simulink model "Quadruple_Tank_Simu_Model"  (R2021b)
settings: Solver=VariableStepAuto  StartTime=0.0  StopTime=300  FixedStep=1  RelTol=1e-3
values from neighbouring files (symbols this model uses):
  a1 = 0.17795237427    [Dados_Tanques.mat]    (also in double_tank_simu.m)
  A1 = 15.5179165474    [Dados_Tanques.mat]    (also in double_tank_simu.m)
  a2 = 0.17795237427    [Dados_Tanques.mat]    (also in double_tank_simu.m)
  A2 = 15.5179165474    [Dados_Tanques.mat]    (also in double_tank_simu.m)
  g = 981    [Dados_Tanques.mat]    (also in double_tank_simu.m)
  x1eq = 15    [Dados_Tanques.mat]    (also in double_tank_simu.m = (1/(2*g))*((km*ueq)/a1)^2)
  x2eq = 15    [Dados_Tanques.mat]    (also in double_tank_simu.m)
undefined symbols (not defined in the file or in its folder): a3, A3, a4, A4, k1, k2, q1, q2, u1eq, u2eq, x3eq, x4eq
libraries: instrumentlib x2
settings Model: Creator=mathe  LastModifiedBy=mathe

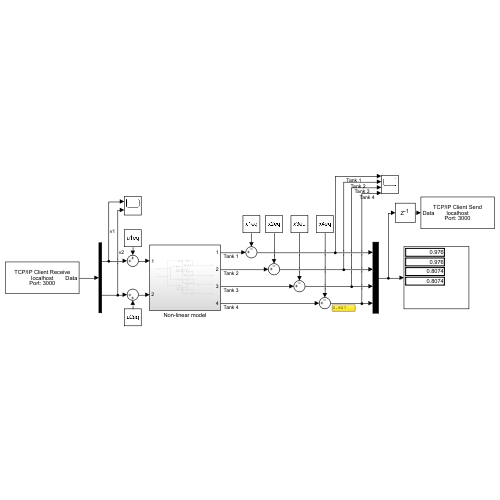
[thumbnail: Simulink's stored preview of the top-level diagram]
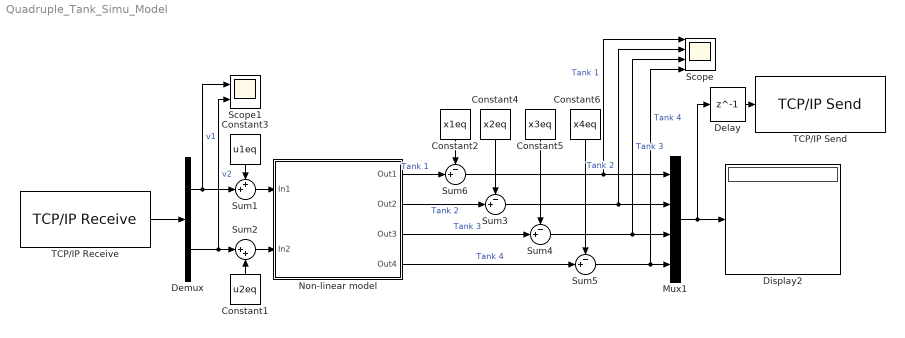
== system Quadruple_Tank_Simu_Model ==
  Constant1 : Constant  Value=u2eq
  Constant2 : Constant  Value=x1eq
  Constant3 : Constant  Value=u1eq
  Constant4 : Constant  Value=x2eq
  Constant5 : Constant  Value=x3eq
  Constant6 : Constant  Value=x4eq
  Delay : Delay  DelayLength=1  InitialCondition=0
  Demux : Demux  Outputs=2
  Display2 : Display
  Mux1 : Mux
  Non-linear model : Subsystem
  Scope : Scope  NumInputPorts=4
  Scope1 : Scope  NumInputPorts=2
  Sum1 : Sum  Inputs=++|
  Sum2 : Sum  Inputs=|++
  Sum{3..6} (4 alike) : Sum  Inputs=-+|
  TCP/IP Receive : instrumentlib/TCP//IP Receive  Priority=2  Host=localhost  Port=3000  DataSize=[ 2, 1 ]  DataType=double  ASCIIFormatting=%f  Terminator=LF  CustomTerminator=10  ByteOrder=big-endian  EnableBlockingMode=on  Timeout=300  SampleTime=1  SimulateUsing=Interpreted execution
  TCP/IP Send : instrumentlib/TCP//IP Send  Priority=1  Host=localhost  Port=3000  ByteOrder=big-endian  EnableBlockingMode=on  Timeout=300  TransferDelay=off  SimulateUsing=Interpreted execution
  wires:
  Non-linear model/1(Out1) -> Sum6/2  "Tank 1"
  Constant3/1 -> Sum1/1
  Sum1/1 -> Non-linear model/1(In1)
  Sum2/1 -> Non-linear model/2(In2)
  Constant1/1 -> Sum2/2
  Sum6/1 -> Scope/1, Mux1/1  "Tank 1"
  Constant2/1 -> Sum6/1
  Sum3/1 -> Scope/2, Mux1/2  "Tank 2"
  Non-linear model/2(Out2) -> Sum3/2  "Tank 2"
  Constant4/1 -> Sum3/1
  Sum5/1 -> Scope/4, Mux1/4  "Tank 4"
  Non-linear model/4(Out4) -> Sum5/2  "Tank 4"
  Non-linear model/3(Out3) -> Sum4/2  "Tank 3"
  Sum4/1 -> Scope/3, Mux1/3  "Tank 3"
  Constant5/1 -> Sum4/1
  Constant6/1 -> Sum5/1
  Demux/1 -> Scope1/1, Sum1/2  "v1"
  Demux/2 -> Scope1/2, Sum2/1  "v2"
  Mux1/1 -> Delay/1, Display2/1
  TCP/IP Receive/1 -> Demux/1
  Delay/1 -> TCP/IP Send/1

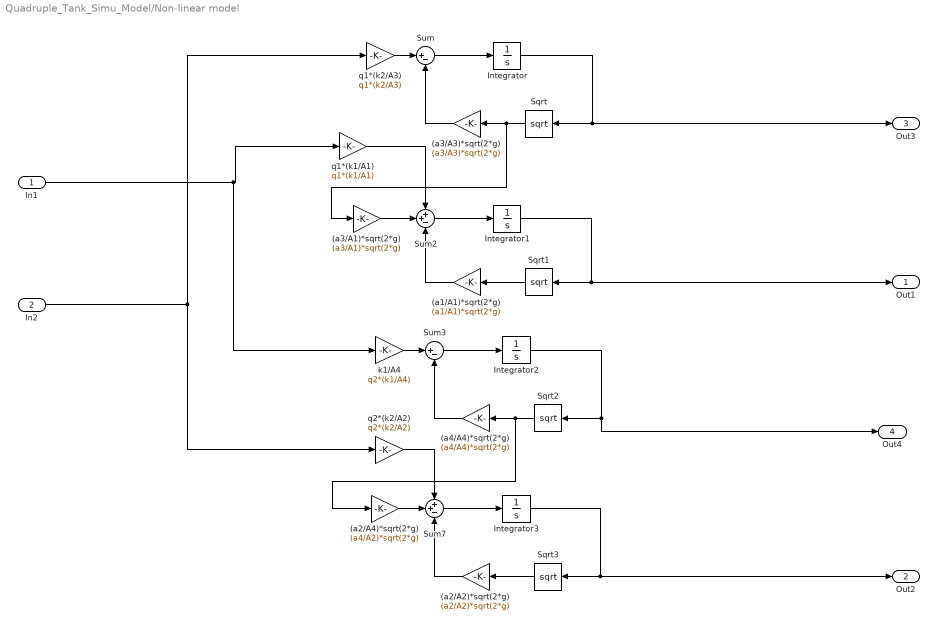
== system Quadruple_Tank_Simu_Model/Non-linear model ==
  In1 : Inport
  In2 : Inport  Port=2
  (a1/A1)*sqrt(2*g) : Gain  Gain=(a1/A1)*sqrt(2*g)
  (a2/A2)*sqrt(2*g) : Gain  Gain=(a2/A2)*sqrt(2*g)
  (a2/A4)*sqrt(2*g) : Gain  Gain=(a4/A2)*sqrt(2*g)
  (a3/A1)*sqrt(2*g) : Gain  Gain=(a3/A1)*sqrt(2*g)
  (a3/A3)*sqrt(2*g) : Gain  Gain=(a3/A3)*sqrt(2*g)
  (a4/A4)*sqrt(2*g) : Gain  Gain=(a4/A4)*sqrt(2*g)
  Integrator : Integrator  InitialCondition=x3eq+1
  Integrator1 : Integrator  InitialCondition=x1eq+1
  Integrator2 : Integrator  InitialCondition=x4eq+1
  Integrator3 : Integrator  InitialCondition=x2eq+1
  Sqrt{,1..3} (4 alike) : Sqrt  SaturateOnIntegerOverflow=on
  Sum : Sum  Inputs=|+-
  Sum2 : Sum  Inputs=++-
  Sum3 : Sum  Inputs=|+-
  Sum7 : Sum  Inputs=++-
  k1/A4 : Gain  Gain=q2*(k1/A4)
  q1*(k1/A1) : Gain  Gain=q1*(k1/A1)
  q1*(k2/A3) : Gain  Gain=q1*(k2/A3)
  q2*(k2/A2) : Gain  Gain=q2*(k2/A2)
  Out1 : Outport
  Out2 : Outport  Port=2
  Out3 : Outport  Port=3
  Out4 : Outport  Port=4
  wires:
  In2/1 -> q2*(k2/A2)/1, q1*(k2/A3)/1
  Integrator3/1 -> Out2/1, Sqrt3/1
  Sqrt2/1 -> (a2/A4)*sqrt(2*g)/1, (a4/A4)*sqrt(2*g)/1
  In1/1 -> k1/A4/1, q1*(k1/A1)/1
  q2*(k2/A2)/1 -> Sum7/1
  (a3/A1)*sqrt(2*g)/1 -> Sum2/2
  Integrator2/1 -> Out4/1, Sqrt2/1
  Sqrt/1 -> (a3/A1)*sqrt(2*g)/1, (a3/A3)*sqrt(2*g)/1
  (a2/A4)*sqrt(2*g)/1 -> Sum7/2
  (a2/A2)*sqrt(2*g)/1 -> Sum7/3
  Sum7/1 -> Integrator3/1
  (a4/A4)*sqrt(2*g)/1 -> Sum3/2
  Integrator1/1 -> Out1/1, Sqrt1/1
  q1*(k2/A3)/1 -> Sum/1
  (a1/A1)*sqrt(2*g)/1 -> Sum2/3
  Sum/1 -> Integrator/1
  Sqrt1/1 -> (a1/A1)*sqrt(2*g)/1
  (a3/A3)*sqrt(2*g)/1 -> Sum/2
  k1/A4/1 -> Sum3/1
  Sqrt3/1 -> (a2/A2)*sqrt(2*g)/1
  Integrator/1 -> Out3/1, Sqrt/1
  Sum3/1 -> Integrator2/1
  Sum2/1 -> Integrator1/1
  q1*(k1/A1)/1 -> Sum2/1
